simulink model "control"  (R2023a)
settings: Solver=VariableStepAuto  StartTime=0.0  StopTime=10.0  RelTol=1e-3
undefined symbols (not defined in the file): maxDeg
settings Model: Creator=Алексей  LastModifiedBy=Алексей

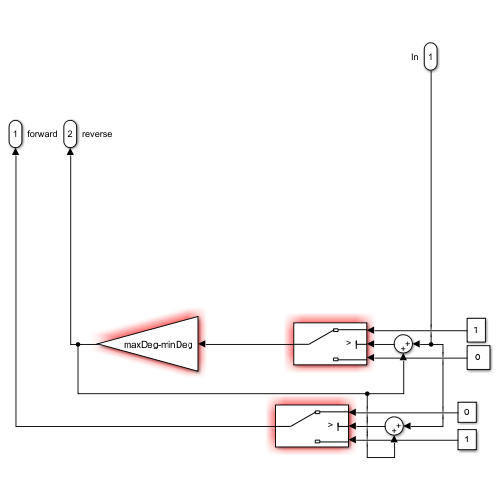
[thumbnail: Simulink's stored preview of the top-level diagram]
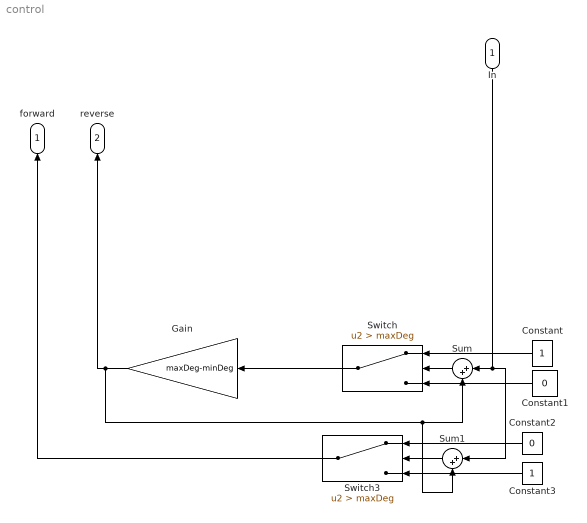
== system control ==
  In : Inport
  Constant : Constant
  Constant1 : Constant  Value=0
  Constant2 : Constant  Value=0
  Constant3 : Constant
  Gain : Gain  Gain=maxDeg-minDeg
  Sum : Sum  Inputs=|++
  Sum1 : Sum  Inputs=|++
  Switch : Switch  Criteria=u2 > Threshold  Threshold=maxDeg  SaturateOnIntegerOverflow=off  InputSameDT=off
  Switch3 : Switch  Criteria=u2 > Threshold  Threshold=maxDeg  SaturateOnIntegerOverflow=off  InputSameDT=off
  forward : Outport
  reverse : Outport  Port=2
  wires:
  Sum1/1 -> Switch3/2
  Constant/1 -> Switch/1
  Switch/1 -> Gain/1
  Gain/1 -> Sum1/2, Sum/2, reverse/1
  Sum/1 -> Switch/2
  Constant1/1 -> Switch/3
  Constant2/1 -> Switch3/1
  Constant3/1 -> Switch3/3
  Switch3/1 -> forward/1
  In/1 -> Sum1/1, Sum/1
